simulink model "p02_PID_FUZZY"  (R2016a)
settings: Solver=VariableStepAuto  StartTime=0.0  StopTime=100  RelTol=1e-3
libraries: fuzblock x1
settings Model: Creator=Administrator  LastModifiedBy=Administrator

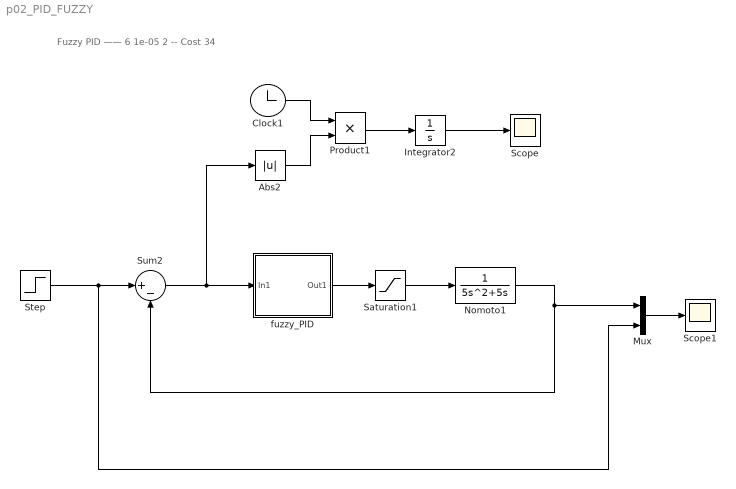
== system p02_PID_FUZZY ==
  note: Fuzzy PID —— 6 1e-05 2 -- Cost 34
  Abs2 : Abs
  Clock1 : Clock
  Integrator2 : Integrator
  Mux : Mux  Inputs=2
  Nomoto1 : TransferFcn  Denominator=[5 5 0]
  Product1 : Product
  Saturation1 : Saturate  UpperLimit=2  LowerLimit=-2
  Scope : Scope
  Scope1 : Scope
  Step : Step  Time=10  SampleTime=0
  Sum2 : Sum  Inputs=|+-
  fuzzy_PID : Subsystem
  wires:
  Integrator2/1 -> Scope/1
  Sum2/1 -> Abs2/1, fuzzy_PID/1(In1)
  Nomoto1/1 -> Sum2/2, Mux/1
  Saturation1/1 -> Nomoto1/1
  fuzzy_PID/1(Out1) -> Saturation1/1
  Clock1/1 -> Product1/1
  Product1/1 -> Integrator2/1
  Abs2/1 -> Product1/2
  Step/1 -> Mux/2, Sum2/1
  Mux/1 -> Scope1/1

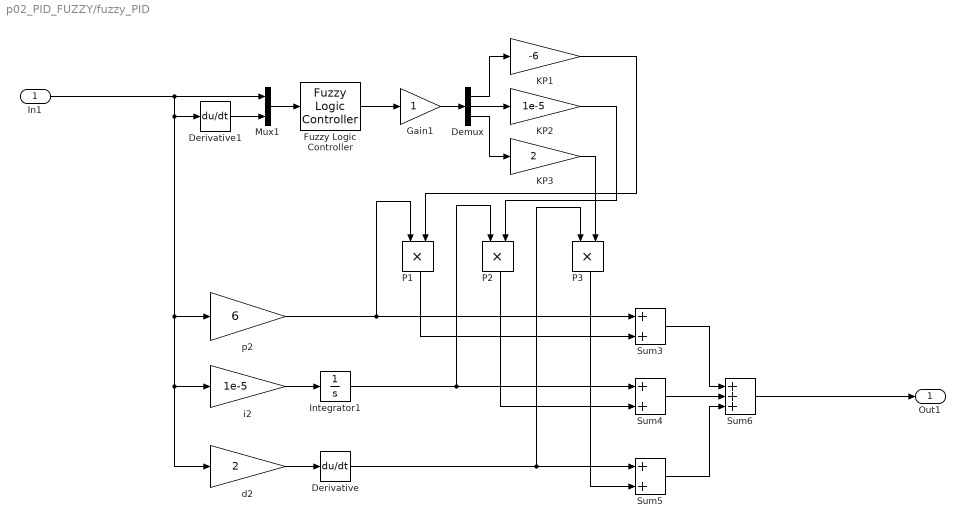
== system p02_PID_FUZZY/fuzzy_PID ==
  In1 : Inport
  Demux : Demux  Outputs=3
  Derivative : Derivative
  Derivative1 : Derivative
  Fuzzy Logic Controller : fuzblock/Fuzzy Logic  Controller  fis='p02_fuzzy_pid.fis'
  Gain1 : Gain
  Integrator1 : Integrator
  KP1 : Gain  Gain=-6
  KP2 : Gain  Gain=1e-5
  KP3 : Gain  Gain=2
  Mux1 : Mux  Inputs=2
  P1 : Product
  P2 : Product
  P3 : Product
  Sum3 : Sum
  Sum4 : Sum
  Sum5 : Sum
  Sum6 : Sum  Inputs=+++
  d2 : Gain  Gain=2
  i2 : Gain  Gain=1e-5
  p2 : Gain  Gain=6
  Out1 : Outport
  wires:
  Demux/2 -> KP2/1
  Mux1/1 -> Fuzzy Logic Controller/1
  Demux/1 -> KP1/1
  In1/1 -> d2/1, i2/1, p2/1, Derivative1/1, Mux1/1
  Derivative1/1 -> Mux1/2
  d2/1 -> Derivative/1
  KP2/1 -> P2/2
  Sum4/1 -> Sum6/2
  Sum5/1 -> Sum6/3
  Sum3/1 -> Sum6/1
  KP1/1 -> P1/2
  Sum6/1 -> Out1/1
  KP3/1 -> P3/2
  i2/1 -> Integrator1/1
  Demux/3 -> KP3/1
  Fuzzy Logic Controller/1 -> Gain1/1
  Gain1/1 -> Demux/1
  p2/1 -> P1/1, Sum3/1
  Integrator1/1 -> Sum4/1, P2/1
  Derivative/1 -> P3/1, Sum5/1
  P1/1 -> Sum3/2
  P2/1 -> Sum4/2
  P3/1 -> Sum5/2
